simulink model "simulink_couple_to_xy"  (R2024b)
settings: Solver=VariableStepAuto  StartTime=0.0  StopTime=100  RelTol=1e-3
values from neighbouring files (symbols this model uses):
  alpha_d_ini = 0    [projet.m]
  alpha_g_ini = 0    [projet.m]
  x0 = 0    [projet.m]
  y0 = 0    [projet.m]
settings Model: Creator=yann  LastModifiedBy=yann

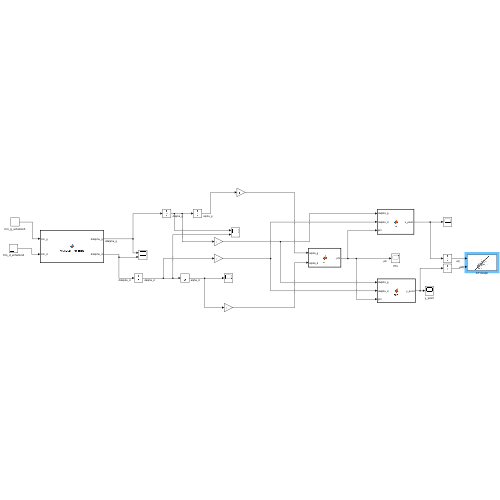
[thumbnail: Simulink's stored preview of the top-level diagram]
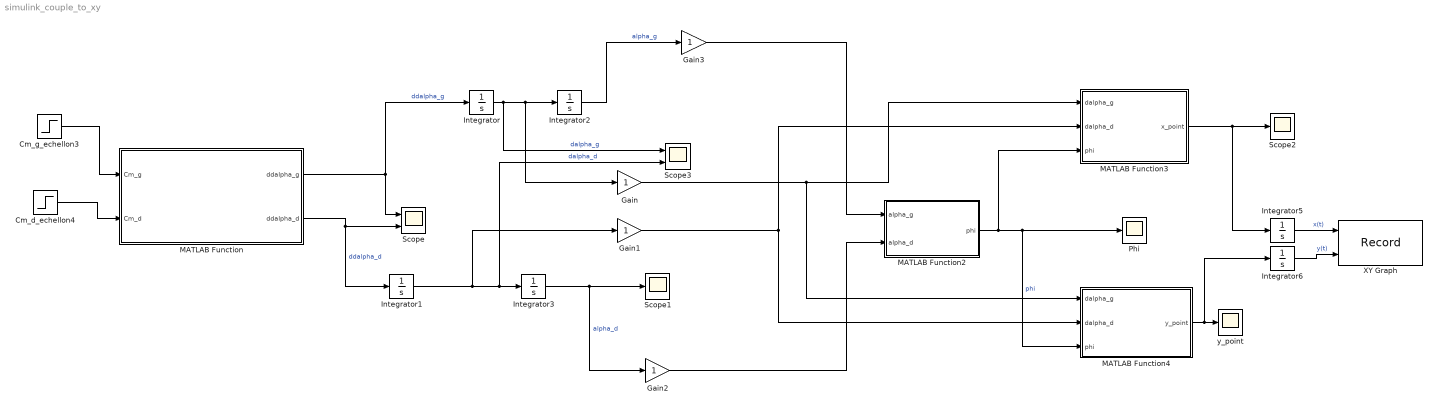
== system simulink_couple_to_xy ==
  Cm_d_echellon4 : Step  Time=0  SampleTime=0
  Cm_g_echellon3 : Step  Time=0  SampleTime=0
  Gain{,1..3} (4 alike) : Gain
  Integrator : Integrator
  Integrator1 : Integrator
  Integrator2 : Integrator  InitialCondition=alpha_g_ini
  Integrator3 : Integrator  InitialCondition=alpha_d_ini
  Integrator5 : Integrator  InitialCondition=x0
  Integrator6 : Integrator  InitialCondition=y0
  MATLAB Function : MATLAB Function  TreatAsAtomicUnit=on
  MATLAB Function2 : MATLAB Function  TreatAsAtomicUnit=on
  MATLAB Function3 : MATLAB Function  TreatAsAtomicUnit=on
  MATLAB Function4 : MATLAB Function  TreatAsAtomicUnit=on
  Phi : Scope
  Scope : Scope  NumInputPorts=2
  Scope1 : Scope
  Scope2 : Scope
  Scope3 : Scope  NumInputPorts=2
  XY Graph : Record  FileSettingsInternal="{\"entries\":[{\"content\":{\"excelSettings\":{\"content\":{},\"type\":\"Streamout.ExcelSettings\"}},\"type\":\"Streamout.FileSettingStorage\",\"uuid\":\"\"}],\"packageUris\":[\"http:\\/\\/schema.mathworks.com\\/mf0\\/streamout_blocks\\/R2020a\"],\"version\":\"1.0\"}"  Layout=[1 1]  SignalsInternal="{\"entries\":[{\"content\":{\"signals\":[{\"content\":{\"blockPath\":[],\"dimensions\":[1],\"domain\":\"\",\"lineColor\":\"#a2142f\",\"plots\":[ 1 ],\"port\":1,\"sid\":[\"\"],\"signalID\":1,\"signalName\":\"x(t)\"},\"type\":\"RecordBlkView.Signal\",\"uuid\":\"\"},{\"content\":{\"blockPath\":[],\"dimensions\":[1],\"domain\":\"\",\"lineColor\":\"#139fff\",\"plots\":[ 1 ],\"port\":2,\"sid\":[\"\"],\"signalID\":2,\"signalName\":\"y(t)\"},\"type\":\"RecordBlkView.Signal\",\"uuid\":\"\"}]},\"type\":\"RecordBlkView.InputSignals\",\"uuid\":\"\"}],\"packageUris\":[\"http:\\/\\/schema.mathworks.com\\/mf0\\/streamout_blocks\\/R2020a\"],\"version\":\"1.0\"}"  VisualizationBindings="{\"xyplotplugin\":{\"info\":[{\"series\":[{\"bindingParametersList\":[{\"parameter\":\"X-Axis\",\"signalID\":1,\"signalName\":\"x(t)\"},{\"parameter\":\"Y-Axis\",\"signalID\":2,\"signalName\":\"y(t)\"}],\"seriesID\":0}],\"subplotID\":1}]}}"  CompatibilityTag=XY
  y_point : Scope
  wires:
  MATLAB Function/1(ddalpha_g) -> Integrator/1, Scope/1  "ddalpha_g"
  Integrator/1 -> Scope3/1, Gain/1, Integrator2/1  "dalpha_g"
  MATLAB Function/2(ddalpha_d) -> Integrator1/1, Scope/2  "ddalpha_d"
  Integrator1/1 -> Gain1/1, Scope3/2, Integrator3/1  "dalpha_d"
  Integrator2/1 -> Gain3/1  "alpha_g"
  Integrator3/1 -> Gain2/1, Scope1/1  "alpha_d"
  Integrator5/1 -> XY Graph/1  "x(t)"
  MATLAB Function2/1(phi) -> MATLAB Function3/3(phi), MATLAB Function4/3(phi), Phi/1  "phi"
  MATLAB Function4/1(y_point) -> Integrator6/1, y_point/1
  MATLAB Function3/1(x_point) -> Integrator5/1, Scope2/1
  Integrator6/1 -> XY Graph/2  "y(t)"
  Gain1/1 -> MATLAB Function4/2(dalpha_d), MATLAB Function3/2(dalpha_d)
  Gain/1 -> MATLAB Function4/1(dalpha_g), MATLAB Function3/1(dalpha_g)
  Gain3/1 -> MATLAB Function2/1(alpha_g)
  Gain2/1 -> MATLAB Function2/2(alpha_d)
  Cm_d_echellon4/1 -> MATLAB Function/2(Cm_d)
  Cm_g_echellon3/1 -> MATLAB Function/1(Cm_g)

== matlab function simulink_couple_to_xy/MATLAB Function ==
  data: ddalpha_g output; Cm_g input; Cm_d input; ddalpha_d output
function [ddalpha_g,ddalpha_d] = MATLAB_Function(Cm_g, Cm_d)
h=2;
l=15e-2;
L=2*l;
R=10e-2;
m_B=750;
e=2e-2;
rho=1200;
mr=300e-3;
I = m_B * (L*2 + h*2) / 12;
Ie = rho*R^2;
I_orth =1/4*mr*R*2+1/10*mr*e*2;

K=2*(0.5*I+I_orth)*(R^2)/(4*l^2);


ddalpha_d = ((-K*Cm_g)/(K+Ie+0.5*m_B*R^2)+Cm_d)/(K+Ie+0.5*m_B*R^2) ;
ddalpha_d=ddalpha_d/(1-((K^2)/(K+Ie+0.5*m_B*R^2))/(K+Ie+0.5*m_B*R^2));

ddalpha_g = (-2*(0.5*I + I_orth)*((R^2)/(4*l^2))*ddalpha_d+Cm_g);
ddalpha_g=ddalpha_g/(2*(0.5*I+I_orth)*((R^2)/(4*l^2))+Ie+0.5*m_B*R^2);
end

== matlab function simulink_couple_to_xy/MATLAB Function2 ==
  data: alpha_g input; phi output; alpha_d input
function phi = fcn(alpha_g, alpha_d)
    R=10e-2;
    l=15e-2;
    

    phi = (-R /(2*l)) *(alpha_g+alpha_d); 
end

== matlab function simulink_couple_to_xy/MATLAB Function3 ==
  data: dalpha_g input; x_point output; dalpha_d input; phi input
function x_point = fcn(dalpha_g,dalpha_d,phi)
    R=0.1;
    x_point = (R/2)*((dalpha_g+dalpha_d)*cos(phi)+(dalpha_d-dalpha_g)*sin(phi));
end

== matlab function simulink_couple_to_xy/MATLAB Function4 ==
  data: dalpha_g input; y_point output; dalpha_d input; phi input
function y_point = fcn(dalpha_g,dalpha_d,phi)
    R=0.1;
    y_point = (R/2)*((dalpha_g-dalpha_d)*cos(phi)+(dalpha_d+dalpha_g)*sin(phi));
end
